simulink model "combinedTxRx_ADIDMA"  (R2019b)
settings: Solver=FixedStepDiscrete  StartTime=0.0  StopTime=10.0  RelTol=1e-3
InitFcn:
  | modelSettings
undefined symbols (not defined in the file): RadioSampleRate
libraries: simulink x4, dspsigops x4, RxTxFixedPointLibrary_noscopes x2, commsource2 x1, commfilt2 x1
settings Model: Creator=tcollins  LastModifiedBy=bhisma
settings DataIOCC: ReturnWorkspaceOutputs=off
settings OptimizationCC: BlockReduction=off  ConditionallyExecuteInputs=off  DefaultParameterBehavior=Inlined
settings DebuggingCC: AlgebraicLoopMsg=error  SingleTaskRateTransMsg=error  ArithmeticOperatorsInVariantConditions=warning
settings HardwareCC: ProdBitPerPointer=32  ProdBitPerSizeT=32  ProdBitPerPtrDiffT=32  ProdLargestAtomicFloat=None  ProdIntDivRoundTo=Undefined  ProdEndianess=Unspecified  ProdWordSize=32  ProdHWDeviceType=ASIC/FPGA->ASIC/FPGA  ProdEqTarget=off
settings SFSimCC: SimUseLocalCustomCode=off  CustomCodeUndefinedFunction=UseInterfaceOnly
settings RTWCC: RTWUseLocalCustomCode=off
settings CodeAppCC: StateflowObjectComments=on

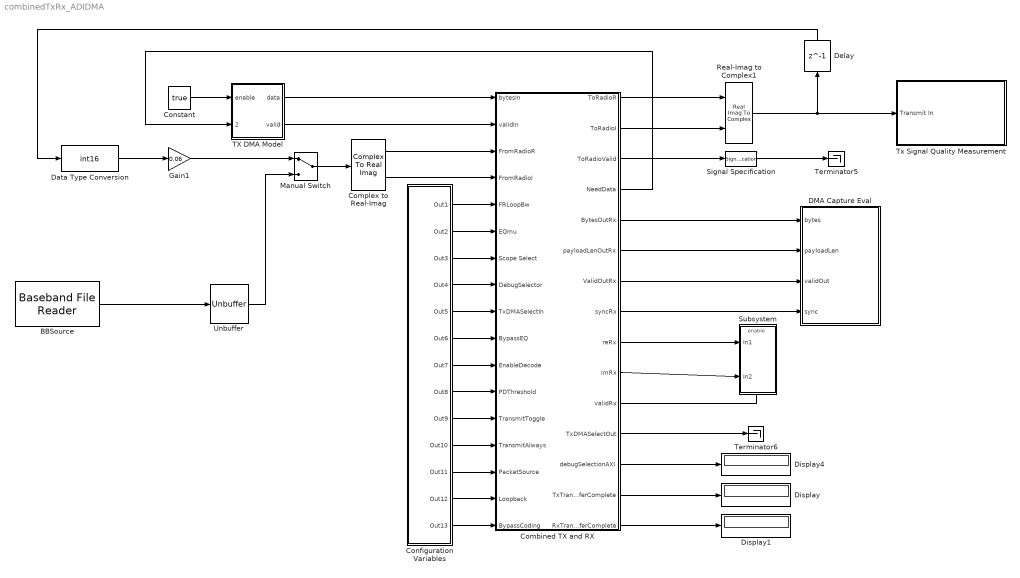
== system combinedTxRx_ADIDMA ==
  BBSource : commsource2/Baseband File Reader  Filename=PlutoCaptureQPSK.bb  InheritSampleTimeFromFile=off  SampleTime=100000/(RadioSampleRate)  SamplesPerFrame=100000  CyclicRepetition=off  FileEndOutputPort=off  SimulateUsing=Interpreted execution
      settings: SourceProductName=Communications Toolbox  SourceProductBaseCode=CM
  Combined TX and RX : Subsystem  TreatAsAtomicUnit=on
  Complex to Real-Imag : ComplexToRealImag
  Configuration Variables : Subsystem
  Constant : Constant  Value=true  SampleTime=-1
  DMA Capture Eval : MATLAB Function  TreatAsAtomicUnit=on
  Data Type Conversion : DataTypeConversion  OutDataTypeStr=int16  ConvertRealWorld=Stored Integer (SI)
  Delay : Delay  DelayLength=1
  Display : Display
  Display1 : Display
  Display4 : Display
  Gain1 : Gain  Gain=0.06  OutDataTypeStr=int16
  Manual Switch : ManualSwitch
  Real-Imag to Complex1 : RealImagToComplex
  Signal Specification : SignalSpecification  SampleTime=1/RadioSampleRate
  Subsystem : Subsystem
  TX DMA Model : Subsystem
  Terminator5 : Terminator
  Terminator6 : Terminator
  Tx Signal Quality Measurement : Subsystem
  Unbuffer : Unbuffer
  wires:
  BBSource/1 -> Unbuffer/1
  Complex to Real-Imag/1 -> Combined TX and RX/3(FromRadioR)
  Complex to Real-Imag/2 -> Combined TX and RX/4(FromRadioI)
  Combined TX and RX/1(ToRadioR) -> Real-Imag to Complex1/1
  Combined TX and RX/2(ToRadioI) -> Real-Imag to Complex1/2
  Combined TX and RX/3(ToRadioValid) -> Signal Specification/1
  Combined TX and RX/5(BytesOutRx) -> DMA Capture Eval/1(bytes)
  Combined TX and RX/6(payloadLenOutRx) -> DMA Capture Eval/2(payloadLen)
  Combined TX and RX/8(syncRx) -> DMA Capture Eval/4(sync)
  Combined TX and RX/11(validRx) -> Subsystem/Enable
  Real-Imag to Complex1/1 -> Delay/1, Tx Signal Quality Measurement/1(Transmit In)
  Configuration Variables/3(Out3) -> Combined TX and RX/7(Scope Select)
  Configuration Variables/1(Out1) -> Combined TX and RX/5(FRLoopBw)
  Configuration Variables/2(Out2) -> Combined TX and RX/6(EQmu)
  Combined TX and RX/7(ValidOutRx) -> DMA Capture Eval/3(validOut)
  Constant/1 -> TX DMA Model/1(enable)
  Combined TX and RX/4(NeedData) -> TX DMA Model/2(enableTx)
  TX DMA Model/1(data) -> Combined TX and RX/1(bytesIn)
  TX DMA Model/2(valid) -> Combined TX and RX/2(validIn)
  Combined TX and RX/12(TxDMASelectOut) -> Terminator6/1
  Combined TX and RX/13(debugSelectionAXI) -> Display4/1
  Configuration Variables/4(Out4) -> Combined TX and RX/8(DebugSelector)
  Configuration Variables/5(Out5) -> Combined TX and RX/9(TxDMASelectIn)
  Signal Specification/1 -> Terminator5/1
  Configuration Variables/6(Out6) -> Combined TX and RX/10(BypassEQ)
  Configuration Variables/7(Out7) -> Combined TX and RX/11(EnableDecode)
  Combined TX and RX/14(TxTransferComplete) -> Display/1
  Delay/1 -> Data Type Conversion/1
  Gain1/1 -> Manual Switch/1
  Manual Switch/1 -> Complex to Real-Imag/1
  Data Type Conversion/1 -> Gain1/1
  Unbuffer/1 -> Manual Switch/2
  Configuration Variables/8(Out8) -> Combined TX and RX/12(PDThreshold)
  Configuration Variables/9(Out9) -> Combined TX and RX/13(TransmitToggle)
  Configuration Variables/10(Out10) -> Combined TX and RX/14(TransmitAlways)
  Configuration Variables/11(Out11) -> Combined TX and RX/15(PacketSource)
  Configuration Variables/12(Out12) -> Combined TX and RX/16(Loopback)
  Configuration Variables/13(Out13) -> Combined TX and RX/17(BypassCoding)
  Combined TX and RX/9(reRx) -> Subsystem/1(In1)
  Combined TX and RX/10(imRx) -> Subsystem/2(In2)
  Combined TX and RX/15(RxTransferComplete) -> Display1/1

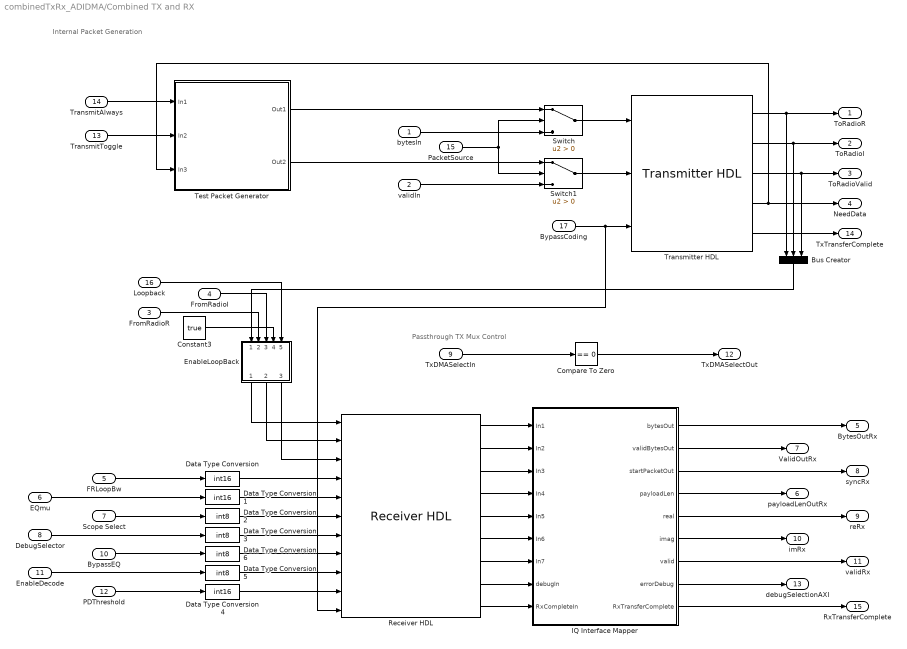
== system combinedTxRx_ADIDMA/Combined TX and RX ==
  note: Passthrough TX Mux Control
  note: Internal Packet Generation
  bytesIn : Inport
  validIn : Inport  Port=2
  FromRadioR : Inport  Port=3
  FromRadioI : Inport  Port=4
  FRLoopBw : Inport  Port=5
  EQmu : Inport  Port=6
  Scope Select : Inport  Port=7
  DebugSelector : Inport  Port=8
  TxDMASelectIn : Inport  Port=9
  BypassEQ : Inport  Port=10
  EnableDecode : Inport  Port=11
  PDThreshold : Inport  Port=12
  TransmitToggle : Inport  Port=13
  TransmitAlways : Inport  Port=14
  PacketSource : Inport  Port=15
  Loopback : Inport  Port=16
  BypassCoding : Inport  Port=17
  Bus Creator : BusCreator  Inputs=3
  Compare To Zero : simulink/Logic and Bit Operations/Compare To Zero  relop===  OutDataTypeStr=boolean
  Constant3 : Constant  Value=true  SampleTime=1/RadioSampleRate
  Data Type Conversion : DataTypeConversion  OutDataTypeStr=int16
  Data Type Conversion1 : DataTypeConversion  OutDataTypeStr=int16
  Data Type Conversion{2..3,5..6} (4 alike) : DataTypeConversion  OutDataTypeStr=int8
  Data Type Conversion4 : DataTypeConversion  OutDataTypeStr=int16
  EnableLoopBack : Subsystem
  IQ Interface Mapper : Subsystem
  Receiver HDL : RxTxFixedPointLibrary_noscopes/Receiver HDL  SystemSampleTime=-1
  Switch : Switch  Criteria=u2 > Threshold
  Switch1 : Switch  Criteria=u2 > Threshold
  Test Packet Generator : Subsystem
  Transmitter HDL : RxTxFixedPointLibrary_noscopes/Transmitter HDL  SystemSampleTime=-1
  ToRadioR : Outport  VectorParamsAs1DForOutWhenUnconnected=off
  ToRadioI : Outport  Port=2  VectorParamsAs1DForOutWhenUnconnected=off
  ToRadioValid : Outport  Port=3  VectorParamsAs1DForOutWhenUnconnected=off
  NeedData : Outport  Port=4  VectorParamsAs1DForOutWhenUnconnected=off
  BytesOutRx : Outport  Port=5  VectorParamsAs1DForOutWhenUnconnected=off
  payloadLenOutRx : Outport  Port=6  VectorParamsAs1DForOutWhenUnconnected=off
  ValidOutRx : Outport  Port=7  VectorParamsAs1DForOutWhenUnconnected=off
  syncRx : Outport  Port=8  VectorParamsAs1DForOutWhenUnconnected=off
  reRx : Outport  Port=9  VectorParamsAs1DForOutWhenUnconnected=off
  imRx : Outport  Port=10  VectorParamsAs1DForOutWhenUnconnected=off
  validRx : Outport  Port=11  VectorParamsAs1DForOutWhenUnconnected=off
  TxDMASelectOut : Outport  Port=12  VectorParamsAs1DForOutWhenUnconnected=off
  debugSelectionAXI : Outport  Port=13  VectorParamsAs1DForOutWhenUnconnected=off
  TxTransferComplete : Outport  Port=14  VectorParamsAs1DForOutWhenUnconnected=off
  RxTransferComplete : Outport  Port=15  VectorParamsAs1DForOutWhenUnconnected=off
  wires:
  Transmitter HDL/2 -> Bus Creator/2, ToRadioI/1
  Transmitter HDL/3 -> ToRadioValid/1, Bus Creator/3
  Transmitter HDL/1 -> ToRadioR/1, Bus Creator/1
  Transmitter HDL/4 -> Test Packet Generator/3(In3), NeedData/1
  FRLoopBw/1 -> Data Type Conversion/1
  EQmu/1 -> Data Type Conversion1/1
  Scope Select/1 -> Data Type Conversion2/1
  TxDMASelectIn/1 -> Compare To Zero/1
  Compare To Zero/1 -> TxDMASelectOut/1
  DebugSelector/1 -> Data Type Conversion3/1
  BypassEQ/1 -> Data Type Conversion6/1
  EnableDecode/1 -> Data Type Conversion5/1
  Receiver HDL/1 -> IQ Interface Mapper/1(In1)
  Receiver HDL/2 -> IQ Interface Mapper/2(In2)
  Receiver HDL/3 -> IQ Interface Mapper/3(In3)
  Receiver HDL/4 -> IQ Interface Mapper/4(In4)
  Receiver HDL/5 -> IQ Interface Mapper/5(In5)
  Receiver HDL/6 -> IQ Interface Mapper/6(In6)
  Receiver HDL/7 -> IQ Interface Mapper/7(In7)
  IQ Interface Mapper/1(bytesOut) -> BytesOutRx/1
  IQ Interface Mapper/2(validBytesOut) -> ValidOutRx/1
  IQ Interface Mapper/3(startPacketOut) -> syncRx/1
  IQ Interface Mapper/4(payloadLen) -> payloadLenOutRx/1
  IQ Interface Mapper/5(real) -> reRx/1
  IQ Interface Mapper/6(imag) -> imRx/1
  IQ Interface Mapper/7(valid) -> validRx/1
  IQ Interface Mapper/8(errorDebug) -> debugSelectionAXI/1
  Transmitter HDL/5 -> TxTransferComplete/1
  PDThreshold/1 -> Data Type Conversion4/1
  Data Type Conversion/1 -> Receiver HDL/4
  Data Type Conversion1/1 -> Receiver HDL/5
  Data Type Conversion2/1 -> Receiver HDL/6
  Data Type Conversion3/1 -> Receiver HDL/7
  Data Type Conversion4/1 -> Receiver HDL/10
  Data Type Conversion5/1 -> Receiver HDL/9
  Data Type Conversion6/1 -> Receiver HDL/8
  PacketSource/1 -> Switch1/2, Switch/2
  EnableLoopBack/1(Out1) -> Receiver HDL/1
  EnableLoopBack/2(Out2) -> Receiver HDL/2
  EnableLoopBack/3(Out3) -> Receiver HDL/3
  FromRadioR/1 -> EnableLoopBack/2(In1)
  FromRadioI/1 -> EnableLoopBack/3(In2)
  Bus Creator/1 -> EnableLoopBack/1(In5)
  Constant3/1 -> EnableLoopBack/4(In3)
  Loopback/1 -> EnableLoopBack/5(In4)
  BypassCoding/1 -> Receiver HDL/11, Transmitter HDL/3
  TransmitAlways/1 -> Test Packet Generator/1(In1)
  TransmitToggle/1 -> Test Packet Generator/2(In2)
  validIn/1 -> Switch1/3
  bytesIn/1 -> Switch/3
  Switch/1 -> Transmitter HDL/1
  Switch1/1 -> Transmitter HDL/2
  Test Packet Generator/1(Out1) -> Switch/1
  Test Packet Generator/2(Out2) -> Switch1/1
  Receiver HDL/8 -> IQ Interface Mapper/8(debugIn)
  Receiver HDL/9 -> IQ Interface Mapper/9(RxCompleteIn)
  IQ Interface Mapper/9(RxTransferComplete) -> RxTransferComplete/1

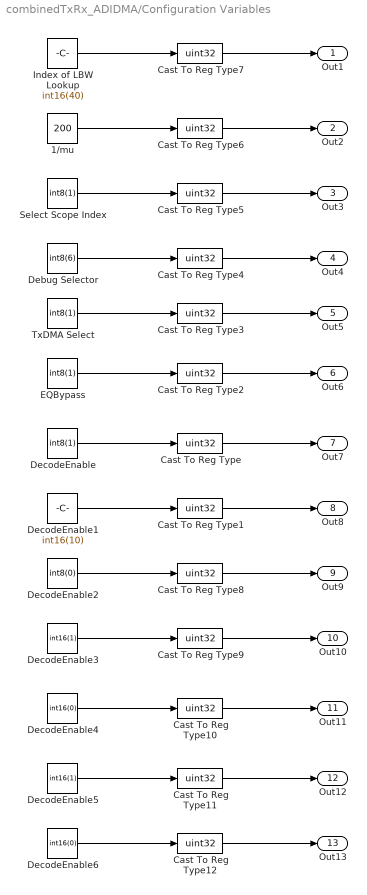
== system combinedTxRx_ADIDMA/Configuration Variables ==
  1/mu : Constant  Value=200  OutDataTypeStr=int16  SampleTime=-1
  Cast To Reg Type{,1..12} (13 alike) : DataTypeConversion  OutDataTypeStr=uint32
  Debug Selector : Constant  Value=int8(6)  SampleTime=1/RadioSampleRate
  DecodeEnable : Constant  Value=int8(1)  SampleTime=1/RadioSampleRate
  DecodeEnable1 : Constant  Value=int16(10)  SampleTime=1/RadioSampleRate
  DecodeEnable2 : Constant  Value=int8(0)  SampleTime=1/RadioSampleRate
  DecodeEnable3 : Constant  Value=int16(1)  SampleTime=1/RadioSampleRate
  DecodeEnable4 : Constant  Value=int16(0)  SampleTime=1/RadioSampleRate
  DecodeEnable5 : Constant  Value=int16(1)  SampleTime=1/RadioSampleRate
  DecodeEnable6 : Constant  Value=int16(0)  SampleTime=1/RadioSampleRate
  EQBypass : Constant  Value=int8(1)  SampleTime=1/RadioSampleRate
  Index of LBW Lookup : Constant  Value=int16(40)  SampleTime=1/RadioSampleRate
  Select Scope Index : Constant  Value=int8(1)  SampleTime=1/RadioSampleRate
  TxDMA Select : Constant  Value=int8(1)  SampleTime=1/RadioSampleRate
  Out1 : Outport  VectorParamsAs1DForOutWhenUnconnected=off
  Out2 : Outport  Port=2  VectorParamsAs1DForOutWhenUnconnected=off
  Out3 : Outport  Port=3  VectorParamsAs1DForOutWhenUnconnected=off
  Out4 : Outport  Port=4  VectorParamsAs1DForOutWhenUnconnected=off
  Out5 : Outport  Port=5  VectorParamsAs1DForOutWhenUnconnected=off
  Out6 : Outport  Port=6  VectorParamsAs1DForOutWhenUnconnected=off
  Out7 : Outport  Port=7  VectorParamsAs1DForOutWhenUnconnected=off
  Out8 : Outport  Port=8  VectorParamsAs1DForOutWhenUnconnected=off
  Out9 : Outport  Port=9  VectorParamsAs1DForOutWhenUnconnected=off
  Out10 : Outport  Port=10  VectorParamsAs1DForOutWhenUnconnected=off
  Out11 : Outport  Port=11  VectorParamsAs1DForOutWhenUnconnected=off
  Out12 : Outport  Port=12  VectorParamsAs1DForOutWhenUnconnected=off
  Out13 : Outport  Port=13  VectorParamsAs1DForOutWhenUnconnected=off
  wires:
  1/mu/1 -> Cast To Reg Type6/1
  Index of LBW Lookup/1 -> Cast To Reg Type7/1
  Select Scope Index/1 -> Cast To Reg Type5/1
  TxDMA Select/1 -> Cast To Reg Type3/1
  Debug Selector/1 -> Cast To Reg Type4/1
  EQBypass/1 -> Cast To Reg Type2/1
  DecodeEnable/1 -> Cast To Reg Type/1
  DecodeEnable1/1 -> Cast To Reg Type1/1
  Cast To Reg Type1/1 -> Out8/1
  Cast To Reg Type/1 -> Out7/1
  Cast To Reg Type2/1 -> Out6/1
  Cast To Reg Type3/1 -> Out5/1
  Cast To Reg Type4/1 -> Out4/1
  Cast To Reg Type5/1 -> Out3/1
  Cast To Reg Type6/1 -> Out2/1
  Cast To Reg Type7/1 -> Out1/1
  DecodeEnable2/1 -> Cast To Reg Type8/1
  DecodeEnable3/1 -> Cast To Reg Type9/1
  Cast To Reg Type9/1 -> Out10/1
  Cast To Reg Type8/1 -> Out9/1
  Cast To Reg Type10/1 -> Out11/1
  DecodeEnable4/1 -> Cast To Reg Type10/1
  DecodeEnable5/1 -> Cast To Reg Type11/1
  Cast To Reg Type11/1 -> Out12/1
  DecodeEnable6/1 -> Cast To Reg Type12/1
  Cast To Reg Type12/1 -> Out13/1

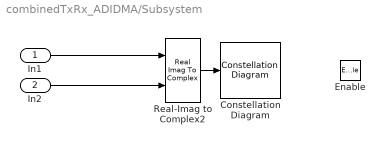
== system combinedTxRx_ADIDMA/Subsystem ==
  In1 : Inport
  In2 : Inport  Port=2
  Enable : EnablePort
  Constellation Diagram : ConstellationDiagram
  Real-Imag to Complex2 : RealImagToComplex
  wires:
  Real-Imag to Complex2/1 -> Constellation Diagram/1
  In1/1 -> Real-Imag to Complex2/1
  In2/1 -> Real-Imag to Complex2/2

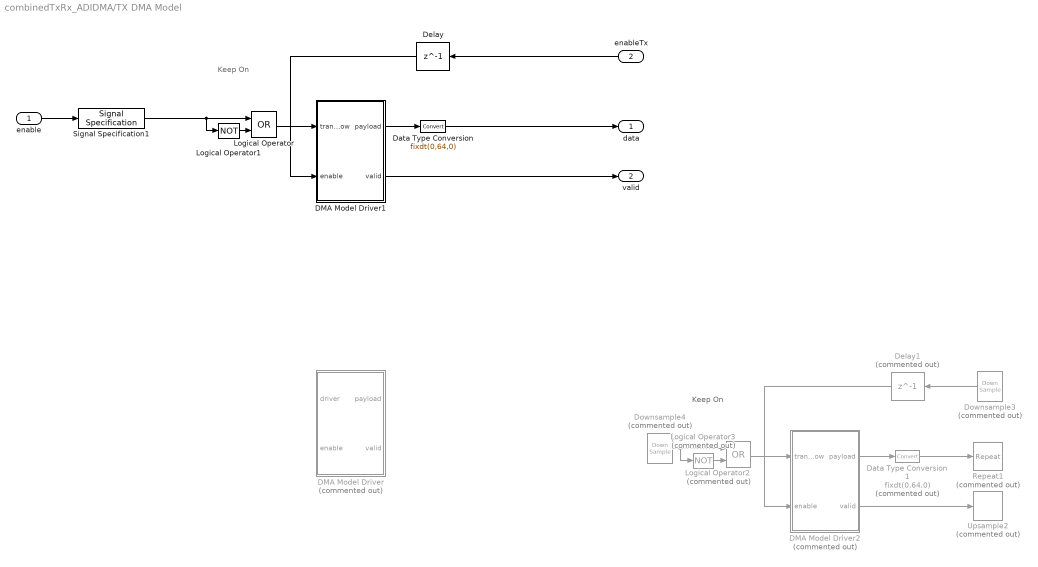
== system combinedTxRx_ADIDMA/TX DMA Model ==
  note: Keep On
  note: Keep On
  enable : Inport
  enableTx : Inport  Port=2
  DMA Model Driver : MATLAB Function  Commented=on  TreatAsAtomicUnit=on
  DMA Model Driver1 : MATLAB Function  TreatAsAtomicUnit=on
  DMA Model Driver2 : MATLAB Function  Commented=on  TreatAsAtomicUnit=on
  Data Type Conversion : DataTypeConversion  OutDataTypeStr=fixdt(0,64,0)
  Data Type Conversion1 : DataTypeConversion  Commented=on  OutDataTypeStr=fixdt(0,64,0)
  Delay : Delay  DelayLength=1
  Delay1 : Delay  Commented=on  DelayLength=1
  Downsample3 : DownSample  Commented=on  N=4  RateOptions=Allow multirate processing
  Downsample4 : DownSample  Commented=on  N=4  RateOptions=Allow multirate processing
  Logical Operator : Logic  Operator=OR  AllPortsSameDT=off  OutDataTypeStr=boolean
  Logical Operator1 : Logic  Operator=NOT  AllPortsSameDT=off  OutDataTypeStr=boolean
  Logical Operator2 : Logic  Commented=on  Operator=OR  AllPortsSameDT=off  OutDataTypeStr=boolean
  Logical Operator3 : Logic  Commented=on  Operator=NOT  AllPortsSameDT=off  OutDataTypeStr=boolean
  Repeat1 : dspsigops/Repeat  Commented=on  N=4  InputProcessing=Columns as channels (frame based)  RateOptions=Allow multirate processing  ic=0  mode=Unused parameter value
      settings: SourceProductName=DSP System Toolbox
  Signal Specification1 : SignalSpecification  OutDataTypeStr=boolean  SampleTime=1e-6
  Upsample2 : dspsigops/Upsample  Commented=on  N=4  phase=0  RateOptions=Allow multirate processing  ic=0  mode=Unused parameter value
  data : Outport  VectorParamsAs1DForOutWhenUnconnected=off
  valid : Outport  Port=2  VectorParamsAs1DForOutWhenUnconnected=off
  wires:
  Signal Specification1/1 -> Logical Operator/1, Logical Operator1/1
  Logical Operator/1 -> DMA Model Driver1/1(transmitNow)
  DMA Model Driver1/2(valid) -> valid/1
  enableTx/1 -> Delay/1
  Delay/1 -> DMA Model Driver1/2(enable)
  Logical Operator1/1 -> Logical Operator/2
  DMA Model Driver1/1(payload) -> Data Type Conversion/1
  enable/1 -> Signal Specification1/1
  Data Type Conversion/1 -> data/1
  DMA Model Driver2/1(payload) -> Data Type Conversion1/1
  Downsample3/1 -> Delay1/1
  Logical Operator3/1 -> Logical Operator2/2
  Delay1/1 -> DMA Model Driver2/2(enable)
  Logical Operator2/1 -> DMA Model Driver2/1(transmitNow)
  Downsample4/1 -> Logical Operator2/1, Logical Operator3/1
  DMA Model Driver2/2(valid) -> Upsample2/1
  Data Type Conversion1/1 -> Repeat1/1

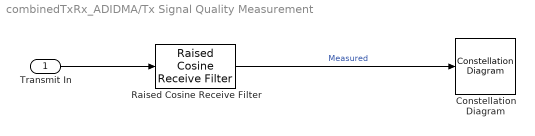
== system combinedTxRx_ADIDMA/Tx Signal Quality Measurement ==
  Transmit In : Inport
  Constellation Diagram : ConstellationDiagram
  Raised Cosine Receive Filter : commfilt2/Raised Cosine Receive Filter  filtType=Square root  R=0.5  filtSpan=8  N=4  downFactor=4  downOffset=0  filterGain=1  RateOptions=Allow multirate processing  framing=Mute  checkCoeff=off  variableName=rcRxFilt  currentFiltSpan=8  D=(8)/2  inputOffset=0  sampMode=Mute  saveAsFlag=0  rateMode=Downsampling  checkGain=Normalized  launchFVT=on  roundingMode=Floor  overflowMode=off  coeffDataTypeStr=Inherit: Same word length as input  coeffMin=[]  coeffMax=[]  coeffLastDataTypeStr=Inherit: Same word length as input  accumDataTypeStr=Inherit: Same as product output  accumLastDataTypeStr=Inherit: Same as product output  outputDataTypeStr=Inherit: Same as accumulator  outputMin=[]  outputMax=[]  outputLastDataTypeStr=Inherit: Same as accumulator
      settings: SourceProductName=Communications Toolbox
  wires:
  Transmit In/1 -> Raised Cosine Receive Filter/1
  Raised Cosine Receive Filter/1 -> Constellation Diagram/1  "Measured"

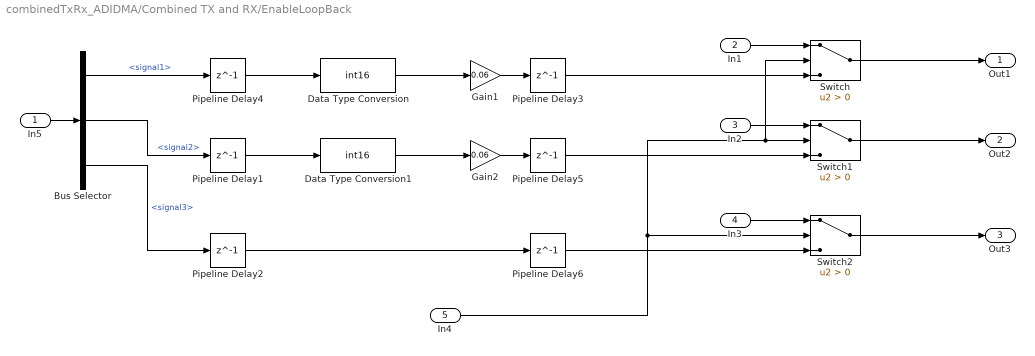
== system combinedTxRx_ADIDMA/Combined TX and RX/EnableLoopBack ==
  In5 : Inport
  In1 : Inport  Port=2
  In2 : Inport  Port=3
  In3 : Inport  Port=4
  In4 : Inport  Port=5
  Bus Selector : BusSelector  OutputSignals=signal1,signal2,signal3
  Data Type Conversion : DataTypeConversion  OutDataTypeStr=int16  ConvertRealWorld=Stored Integer (SI)
  Data Type Conversion1 : DataTypeConversion  OutDataTypeStr=int16  ConvertRealWorld=Stored Integer (SI)
  Gain1 : Gain  Gain=0.06  OutDataTypeStr=int16  SaturateOnIntegerOverflow=on
  Gain2 : Gain  Gain=0.06  OutDataTypeStr=int16  SaturateOnIntegerOverflow=on
  Pipeline Delay{1..6} (6 alike) : Delay  DelayLength=1
  Switch : Switch  Criteria=u2 > Threshold
  Switch1 : Switch  Criteria=u2 > Threshold
  Switch2 : Switch  Criteria=u2 > Threshold
  Out1 : Outport  VectorParamsAs1DForOutWhenUnconnected=off
  Out2 : Outport  Port=2  VectorParamsAs1DForOutWhenUnconnected=off
  Out3 : Outport  Port=3  VectorParamsAs1DForOutWhenUnconnected=off
  wires:
  Switch1/1 -> Out2/1
  Switch2/1 -> Out3/1
  Switch/1 -> Out1/1
  In4/1 -> Switch/2, Switch1/2, Switch2/2
  Pipeline Delay4/1 -> Data Type Conversion/1
  Pipeline Delay1/1 -> Data Type Conversion1/1
  Pipeline Delay2/1 -> Pipeline Delay6/1
  In5/1 -> Bus Selector/1
  Bus Selector/1 -> Pipeline Delay4/1  "<signal1>"
  Bus Selector/2 -> Pipeline Delay1/1  "<signal2>"
  Bus Selector/3 -> Pipeline Delay2/1  "<signal3>"
  Data Type Conversion/1 -> Gain1/1
  Gain1/1 -> Pipeline Delay3/1
  Data Type Conversion1/1 -> Gain2/1
  Gain2/1 -> Pipeline Delay5/1
  In1/1 -> Switch/1
  Pipeline Delay3/1 -> Switch/3
  In2/1 -> Switch1/1
  Pipeline Delay5/1 -> Switch1/3
  In3/1 -> Switch2/1
  Pipeline Delay6/1 -> Switch2/3

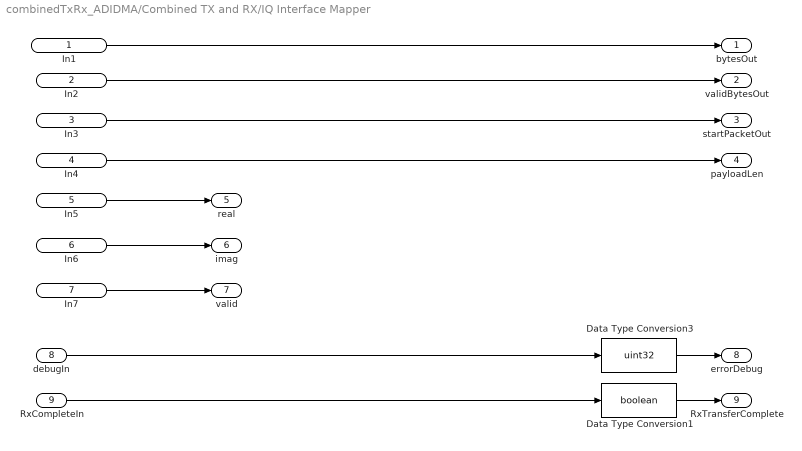
== system combinedTxRx_ADIDMA/Combined TX and RX/IQ Interface Mapper ==
  In1 : Inport
  In2 : Inport  Port=2
  In3 : Inport  Port=3
  In4 : Inport  Port=4
  In5 : Inport  Port=5
  In6 : Inport  Port=6
  In7 : Inport  Port=7
  debugIn : Inport  Port=8
  RxCompleteIn : Inport  Port=9
  Data Type Conversion1 : DataTypeConversion  OutDataTypeStr=boolean
  Data Type Conversion3 : DataTypeConversion  OutDataTypeStr=uint32
  bytesOut : Outport  VectorParamsAs1DForOutWhenUnconnected=off
  validBytesOut : Outport  Port=2  VectorParamsAs1DForOutWhenUnconnected=off
  startPacketOut : Outport  Port=3  VectorParamsAs1DForOutWhenUnconnected=off
  payloadLen : Outport  Port=4  VectorParamsAs1DForOutWhenUnconnected=off
  real : Outport  Port=5  VectorParamsAs1DForOutWhenUnconnected=off
  imag : Outport  Port=6  VectorParamsAs1DForOutWhenUnconnected=off
  valid : Outport  Port=7  VectorParamsAs1DForOutWhenUnconnected=off
  errorDebug : Outport  Port=8  VectorParamsAs1DForOutWhenUnconnected=off
  RxTransferComplete : Outport  Port=9  VectorParamsAs1DForOutWhenUnconnected=off
  wires:
  In2/1 -> validBytesOut/1
  In4/1 -> payloadLen/1
  In7/1 -> valid/1
  debugIn/1 -> Data Type Conversion3/1
  In1/1 -> bytesOut/1
  In3/1 -> startPacketOut/1
  In5/1 -> real/1
  In6/1 -> imag/1
  Data Type Conversion3/1 -> errorDebug/1
  RxCompleteIn/1 -> Data Type Conversion1/1
  Data Type Conversion1/1 -> RxTransferComplete/1

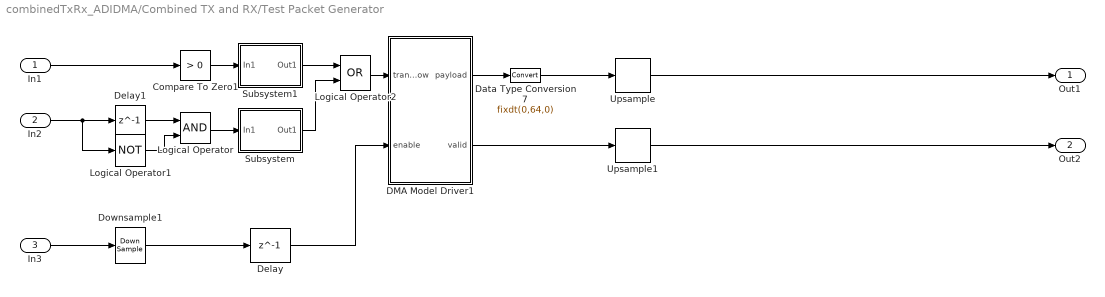
== system combinedTxRx_ADIDMA/Combined TX and RX/Test Packet Generator ==
  In1 : Inport
  In2 : Inport  Port=2
  In3 : Inport  Port=3
  Compare To Zero1 : simulink/Logic and Bit Operations/Compare To Zero  relop=>  OutDataTypeStr=boolean
  DMA Model Driver1 : MATLAB Function  TreatAsAtomicUnit=on
  Data Type Conversion7 : DataTypeConversion  OutDataTypeStr=fixdt(0,64,0)
  Delay : Delay  DelayLength=1
  Delay1 : Delay  DelayLength=1
  Downsample1 : DownSample  N=4  RateOptions=Allow multirate processing
  Logical Operator : Logic  AllPortsSameDT=off  OutDataTypeStr=boolean
  Logical Operator1 : Logic  Operator=NOT  AllPortsSameDT=off  OutDataTypeStr=boolean
  Logical Operator2 : Logic  Operator=OR  AllPortsSameDT=off  OutDataTypeStr=boolean
  Subsystem : Subsystem
  Subsystem1 : Subsystem
  Upsample : dspsigops/Upsample  N=4  phase=0  RateOptions=Allow multirate processing  ic=0  mode=Unused parameter value
  Upsample1 : dspsigops/Upsample  N=4  phase=0  RateOptions=Allow multirate processing  ic=0  mode=Unused parameter value
  Out1 : Outport  VectorParamsAs1DForOutWhenUnconnected=off
  Out2 : Outport  Port=2  VectorParamsAs1DForOutWhenUnconnected=off
  wires:
  In1/1 -> Compare To Zero1/1
  Subsystem/1(Out1) -> Logical Operator2/2
  Logical Operator1/1 -> Logical Operator/2
  DMA Model Driver1/1(payload) -> Data Type Conversion7/1
  Downsample1/1 -> Delay/1
  Delay1/1 -> Logical Operator/1
  Logical Operator/1 -> Subsystem/1(In1)
  Logical Operator2/1 -> DMA Model Driver1/1(transmitNow)
  Subsystem1/1(Out1) -> Logical Operator2/1
  In2/1 -> Logical Operator1/1, Delay1/1
  DMA Model Driver1/2(valid) -> Upsample1/1
  Data Type Conversion7/1 -> Upsample/1
  Compare To Zero1/1 -> Subsystem1/1(In1)
  Upsample1/1 -> Out2/1
  Upsample/1 -> Out1/1
  Delay/1 -> DMA Model Driver1/2(enable)
  In3/1 -> Downsample1/1

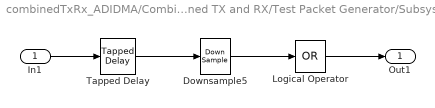
== system combinedTxRx_ADIDMA/Combined TX and RX/Test Packet Generator/Subsystem ==
  In1 : Inport
  Downsample5 : DownSample  N=4  RateOptions=Allow multirate processing
  Logical Operator : Logic  Operator=OR  Inputs=1  AllPortsSameDT=off  OutDataTypeStr=boolean
  Tapped Delay : simulink/Discrete/Tapped Delay  vinit=0.0  samptime=-1  NumDelays=3  DelayOrder=Oldest  includeCurrent=on
  Out1 : Outport  VectorParamsAs1DForOutWhenUnconnected=off
  wires:
  Logical Operator/1 -> Out1/1
  Downsample5/1 -> Logical Operator/1
  Tapped Delay/1 -> Downsample5/1
  In1/1 -> Tapped Delay/1

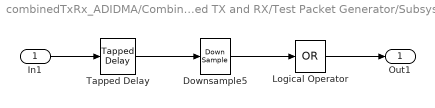
== system combinedTxRx_ADIDMA/Combined TX and RX/Test Packet Generator/Subsystem1 ==
  In1 : Inport
  Downsample5 : DownSample  N=4  RateOptions=Allow multirate processing
  Logical Operator : Logic  Operator=OR  Inputs=1  AllPortsSameDT=off  OutDataTypeStr=boolean
  Tapped Delay : simulink/Discrete/Tapped Delay  vinit=0.0  samptime=-1  NumDelays=3  DelayOrder=Oldest  includeCurrent=on
  Out1 : Outport  VectorParamsAs1DForOutWhenUnconnected=off
  wires:
  Logical Operator/1 -> Out1/1
  Downsample5/1 -> Logical Operator/1
  Tapped Delay/1 -> Downsample5/1
  In1/1 -> Tapped Delay/1

== matlab function combinedTxRx_ADIDMA/Combined TX and RX/Test Packet Generator/DMA Model Driver1 ==
  data: transmitNow input; payload output; valid output boolean; enable input
function [payload,valid] = fcn(transmitNow, enable)
%#codegen

persistent indx mode pSize counter msg payloadIndx transmitNext

if isempty(indx)
    msg = fi(int8('Hello World 0'),0,64,0);
    pSize = fi(length('Hello World 0')*8,0,64,0); % Size in bytes (Must be multiple of 32 bits) cannot exceed uint16 max
    indx = pSize;
    mode = int8(0);
    counter = fi(0,0,64,0);
    payloadIndx = uint8(0);
    transmitNext = false;
end

%% Make default MSG
% Constant

% Update packet count
%msg(uint8(13)) = counter + fi(48,0,64,0);
setting = pSize;

%% Output MSG
if enable
    valid = true;
    switch mode
        case int8(0) % Fresh packet start
            if transmitNow || transmitNext
                pSize = fi(setting,0,64,0);
                payload = fi(setting,0,64,0);%Upper bits
                mode = int8(1);
                payloadIndx = uint8(0);
                indx = fi(0,0,64,0);
                transmitNext = false; % Reset
                %fprintf('(TX) Sending new packet with length: %u\n',uint64(pSize));
            else
                payload = fi(setting,0,64,0);%Upper bits
                valid = false;
            end
        otherwise
            if transmitNow
                transmitNext = true;
            end
            indx = fi(indx + fi(8,0,64,0),0,64,0);
            payloadIndx = payloadIndx + uint8(1);
            payload = msg(payloadIndx);
            if indx == pSize % reached end of frame
                mode = int8(0);
                payloadIndx = uint8(0);
                if counter==fi(9,0,64,0)
                    counter = fi(0,0,64,0);
                else
                    counter = fi(counter + fi(1,0,64,0),0,64,0);
                end
            end
    end
else
    if transmitNow
        transmitNext = true;
    end
    valid = false;
    payload = fi(0,0,64,0);
end

== matlab function combinedTxRx_ADIDMA/DMA Capture Eval ==
  data: bytes input; payloadLen input; validOut input; sync input
function fcn(bytes, payloadLen, validOut, sync)

persistent frameBuffer byteCounter fullPayloadBits

bitsInPack = 64;

if isempty(frameBuffer)
    maxFrameBits = (2^16)*8;
    frameBuffer = false(maxFrameBits,1);
    byteCounter = 0;
    fullPayloadBits = uint16(0);
end

if validOut
    if sync
        byteCounter = bitsInPack;
        frameBuffer(1:byteCounter) = bitget(bytes,1:bitsInPack);
        fullPayloadBits = uint16(payloadLen*8);
        
    elseif byteCounter<fullPayloadBits
        frameBuffer(byteCounter+1:byteCounter+bitsInPack) = bitget(bytes,1:bitsInPack);
        byteCounter = byteCounter + bitsInPack;
    else
        if bytes>0
            disp('CRC Error (Outside)');
        else
            disp('Frame passed CRC (Outside)');
            b = frameBuffer(1:byteCounter);
            fprintf('%s\n',char(bi2de(reshape(b,64,832/64).').'));
        end
    end
end

== matlab function combinedTxRx_ADIDMA/TX DMA Model/DMA Model Driver1 ==
  data: transmitNow input; payload output; valid output boolean; enable input
function [payload,valid] = fcn(transmitNow, enable)
%#codegen

persistent indx mode pSize counter msg payloadIndx transmitNext lastpayload

if isempty(indx)
    msg = fi(int8('Hello World X'),0,64,0);
    pSize = fi(length('Hello World X')*8,0,64,0); % Size in bytes (Must be multiple of 32 bits) cannot exceed uint16 max
    indx = pSize;
    mode = int8(0);
    counter = fi(0,0,64,0);
    payloadIndx = uint8(0);
    transmitNext = false;
    lastpayload = fi(0,0,64,0);
end

%% Make default MSG
% Constant

% Update packet count
%msg(uint8(13)) = counter + fi(48,0,64,0);
setting = pSize;

%% Output MSG
if enable
    valid = true;
    switch mode
        case int8(0) % Fresh packet start
            if transmitNow || transmitNext
                pSize = fi(setting,0,64,0);
                payload = fi(setting,0,64,0);%Upper bits
                mode = int8(1);
                payloadIndx = uint8(0);
                indx = fi(0,0,64,0);
                transmitNext = false; % Reset
                %fprintf('(TX) Sending new packet with length: %u\n',uint64(pSize));
            else
                payload = fi(setting,0,64,0);
                valid = false;
            end
        otherwise
            if transmitNow
                transmitNext = true;
            end
            indx = fi(indx + fi(8,0,64,0),0,64,0);
            payloadIndx = payloadIndx + uint8(1);
            payload = msg(payloadIndx);
            if indx == pSize % reached end of frame
                mode = int8(0);
                payloadIndx = uint8(0);
                if counter==fi(9,0,64,0)
                    counter = fi(0,0,64,0);
                else
                    counter = fi(counter + fi(1,0,64,0),0,64,0);
                end
            end
    end
else
    if transmitNow
        transmitNext = true;
    end
    valid = false;
    payload = lastpayload;
end
lastpayload = payload;

== matlab function combinedTxRx_ADIDMA/TX DMA Model/DMA Model Driver2 ==
  data: transmitNow input; payload output; valid output boolean; enable input
function [payload,valid] = fcn(transmitNow, enable)
%#codegen

persistent indx mode pSize counter msg payloadIndx transmitNext

if isempty(indx)
    msg = fi(int8('Hello World 0'),0,64,0);
    pSize = fi(length('Hello World 0')*8,0,64,0); % Size in bytes (Must be multiple of 32 bits) cannot exceed uint16 max
    indx = pSize;
    mode = int8(0);
    counter = fi(0,0,64,0);
    payloadIndx = uint8(0);
    transmitNext = false;
end

%% Make default MSG
% Constant

% Update packet count
%msg(uint8(13)) = counter + fi(48,0,64,0);
setting = pSize;

%% Output MSG
if enable
    valid = true;
    switch mode
        case int8(0) % Fresh packet start
            if transmitNow || transmitNext
                pSize = fi(setting,0,64,0);
                payload = fi(setting,0,64,0);%Upper bits
                mode = int8(1);
                payloadIndx = uint8(0);
                indx = fi(0,0,64,0);
                transmitNext = false; % Reset
                %fprintf('(TX) Sending new packet with length: %u\n',uint64(pSize));
            else
                payload = fi(setting,0,64,0);%Upper bits
                valid = false;
            end
        otherwise
            if transmitNow
                transmitNext = true;
            end
            indx = fi(indx + fi(8,0,64,0),0,64,0);
            payloadIndx = payloadIndx + uint8(1);
            payload = msg(payloadIndx);
            if indx == pSize % reached end of frame
                mode = int8(0);
                payloadIndx = uint8(0);
                if counter==fi(9,0,64,0)
                    counter = fi(0,0,64,0);
                else
                    counter = fi(counter + fi(1,0,64,0),0,64,0);
                end
            end
    end
else
    if transmitNow
        transmitNext = true;
    end
    valid = false;
    payload = fi(0,0,64,0);
end

== matlab function combinedTxRx_ADIDMA/TX DMA Model/DMA Model Driver ==
  data: driver input; payload output; valid output boolean; enable input
function [payload,valid] = fcn(driver, enable)
%#codegen

persistent indx mode

pSize = fi(200,0,64,0); % Size in bytes (Must be multiple of 32 bits) cannot exceed uint16 max
mask = uint16(sum(2.^(0:15)));

if isempty(indx)
    indx = pSize;
    mode = int8(0);
end

% % Randomly dont transmit new data
% if enable && mode == 0
%    enable = randn>1; 
% end

if enable && driver
    valid = true;
    switch mode
        case int8(0) % Fresh packet start
%             disp('New Packet Start');
            payload = fi(pSize,0,64,0);%Upper bits
            mode = int8(1);
            indx = fi(0,0,64,0);
        otherwise%case 2
            indx = fi(indx + fi(8,0,64,0),0,64,0);
            %payload = uint32(sum(2.^[0 2 4 6 8 10 12 14 ]));
            if indx == fi(8,0,64,0)
                payload = fi(0,0,64,0);
            elseif indx == pSize
                payload = fi(uint64(18446744073709551615),0,64,0); % All ones
            else
                payload = fi(uint64(12297829382473034410),0,64,0);%sum(2.^[0:2:14])); % Alternating ones and zeros
            end
            
            if indx == pSize % reached end of frame
                mode = int8(0);
            end
    end
else
    valid = false;
    payload = fi(0,0,64,0);
end
